simulink model "untitled"  (R2021b)
settings: Solver=VariableStepAuto  StartTime=0.0  StopTime=10.0  RelTol=1e-3
settings Model: Creator=401-06  LastModifiedBy=401-06

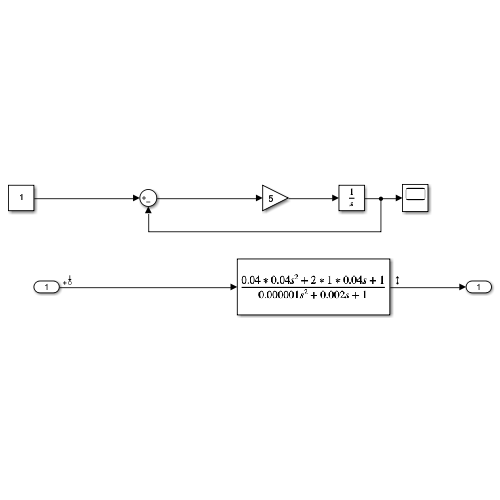
[thumbnail: Simulink's stored preview of the top-level diagram]
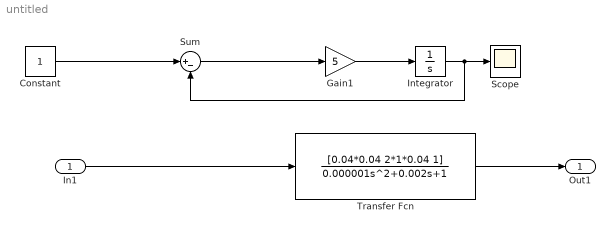
== system untitled ==
  In1 : Inport
  Constant : Constant
  Gain1 : Gain  Gain=5
  Integrator : Integrator
  Scope : Scope
  Sum : Sum  Inputs=|+-
  Transfer Fcn : TransferFcn  Numerator=[0.04*0.04 2*1*0.04 1]  Denominator=[0.000001 0.002 1]
  Out1 : Outport
  wires:
  Constant/1 -> Sum/1
  Sum/1 -> Gain1/1
  Gain1/1 -> Integrator/1
  Integrator/1 -> Sum/2, Scope/1
  In1/1 -> Transfer Fcn/1
  Transfer Fcn/1 -> Out1/1
